simulink model "case3"  (R2024b)
settings: Solver=FixedStepAuto  StartTime=0  StopTime=1  FixedStep=1e-7  RelTol=1e-3
values from neighbouring files (symbols this model uses):
  SG_D_1_D = 0.01056    [IEEE9_case_parameters.m]    (also in case1_parameters.m; case2_parameters.m; case3_parameters.m; case4_parameters.m)
  SG_D_1_EnableSaturation = 0    [IEEE9_case_parameters.m]    (also in case1_parameters.m; case2_parameters.m; case3_parameters.m; case4_parameters.m)
  SG_D_1_f0 = 60    [IEEE9_case_parameters.m]    (also in case1_parameters.m; case2_parameters.m; case3_parameters.m; case4_parameters.m)
  SG_D_1_H = 7.5    [IEEE9_case_parameters.m]    (also in case1_parameters.m; case2_parameters.m; case3_parameters.m; case4_parameters.m)
  SG_D_1_K_A = 20    [IEEE9_case_parameters.m]    (also in case1_parameters.m; case2_parameters.m; case3_parameters.m; case4_parameters.m)
  SG_D_1_K_E = 1.000000e+1    (= 10)    [IEEE9_case_parameters.m]    (also in case1_parameters.m; case2_parameters.m; case3_parameters.m; case4_parameters.m)
  SG_D_1_K_F = 2.363    [IEEE9_case_parameters.m]    (also in case1_parameters.m; case2_parameters.m; case3_parameters.m; case4_parameters.m)
  SG_D_1_K_s = 0.5    [IEEE9_case_parameters.m]    (also in case1_parameters.m = 5; case2_parameters.m = 5; case3_parameters.m = 5; case4_parameters.m = 5)
  SG_D_1_R_a = 0.001088    [IEEE9_case_parameters.m]    (also in case1_parameters.m; case2_parameters.m; case3_parameters.m; case4_parameters.m)
  SG_D_1_S_A = 1    [IEEE9_case_parameters.m]    (also in case1_parameters.m; case2_parameters.m; case3_parameters.m; case4_parameters.m)
  SG_D_1_S_B = 0.103    [IEEE9_case_parameters.m]    (also in case1_parameters.m; case2_parameters.m; case3_parameters.m; case4_parameters.m)
  SG_D_1_S_N = 10.659857    [IEEE9_case_parameters.m]    (also in case1_parameters.m; case2_parameters.m; case3_parameters.m; case4_parameters.m)
  SG_D_1_SpeedPara = 200    [IEEE9_case_parameters.m]    (also in case1_parameters.m; case2_parameters.m; case3_parameters.m; case4_parameters.m)
  SG_D_1_T_0 = 0.720173    [IEEE9_case_parameters.m]    (also in case1_parameters.m = 0.755522; case2_parameters.m = 0.808931; case3_parameters.m = 0.869402; case4_parameters.m = 0.729316)
  SG_D_1_T_1 = 0.3    [IEEE9_case_parameters.m]    (also in case1_parameters.m; case2_parameters.m; case3_parameters.m; case4_parameters.m)
  SG_D_1_T_2 = 0.05    [IEEE9_case_parameters.m]    (also in case1_parameters.m; case2_parameters.m; case3_parameters.m; case4_parameters.m)
  SG_D_1_T_3 = 0.02    [IEEE9_case_parameters.m]    (also in case1_parameters.m; case2_parameters.m; case3_parameters.m; case4_parameters.m)
  SG_D_1_T_4 = 0.005    [IEEE9_case_parameters.m]    (also in case1_parameters.m; case2_parameters.m; case3_parameters.m; case4_parameters.m)
  SG_D_1_T_A = 0.02    [IEEE9_case_parameters.m]    (also in case1_parameters.m; case2_parameters.m; case3_parameters.m; case4_parameters.m)
  SG_D_1_T_dd = 8.000000e+0    (= 8)    [IEEE9_case_parameters.m]    (also in case1_parameters.m; case2_parameters.m; case3_parameters.m; case4_parameters.m)
  SG_D_1_T_ddd = 0.04    [IEEE9_case_parameters.m]    (also in case1_parameters.m; case2_parameters.m; case3_parameters.m; case4_parameters.m)
  SG_D_1_T_E = 0.314    [IEEE9_case_parameters.m]    (also in case1_parameters.m; case2_parameters.m; case3_parameters.m; case4_parameters.m)
  SG_D_1_T_F = 0.35    [IEEE9_case_parameters.m]    (also in case1_parameters.m; case2_parameters.m; case3_parameters.m; case4_parameters.m)
  SG_D_1_T_qd = 0.8    [IEEE9_case_parameters.m]    (also in case1_parameters.m; case2_parameters.m; case3_parameters.m; case4_parameters.m)
  SG_D_1_T_qdd = 0.02    [IEEE9_case_parameters.m]    (also in case1_parameters.m; case2_parameters.m; case3_parameters.m; case4_parameters.m)
  SG_D_1_T_speed = 0.1    [IEEE9_case_parameters.m]    (also in case1_parameters.m = 200; case2_parameters.m = 200; case3_parameters.m = 200; case4_parameters.m = 200)
  SG_D_1_T_w = 0.5    [IEEE9_case_parameters.m]    (also in case1_parameters.m; case2_parameters.m; case3_parameters.m; case4_parameters.m)
  SG_D_1_V_ref = 1.990276    [IEEE9_case_parameters.m]    (also in case1_parameters.m = 2.042296; case2_parameters.m = 2.051388; case3_parameters.m = 2.089584; case4_parameters.m = 2.01845)
  SG_D_1_w_ref = 376.991118    [IEEE9_case_parameters.m]    (also in case1_parameters.m; case2_parameters.m; case3_parameters.m; case4_parameters.m)
  SG_D_1_wb = 6.000000e+1    (= 60)    [IEEE9_case_parameters.m]    (also in case1_parameters.m; case2_parameters.m; case3_parameters.m; case4_parameters.m)
  SG_D_1_x_d = 1.9    [IEEE9_case_parameters.m]    (also in case1_parameters.m; case2_parameters.m; case3_parameters.m; case4_parameters.m)
  SG_D_1_x_dd = 0.302    [IEEE9_case_parameters.m]    (also in case1_parameters.m; case2_parameters.m; case3_parameters.m; case4_parameters.m)
  SG_D_1_x_ddd = 0.204    [IEEE9_case_parameters.m]    (also in case1_parameters.m; case2_parameters.m; case3_parameters.m; case4_parameters.m)
  SG_D_1_x_l = 0.05    [IEEE9_case_parameters.m]    (also in case1_parameters.m; case2_parameters.m; case3_parameters.m; case4_parameters.m)
  SG_D_1_x_q = 1.3    [IEEE9_case_parameters.m]    (also in case1_parameters.m; case2_parameters.m; case3_parameters.m; case4_parameters.m)
  SG_D_1_x_qd = 0.5    [IEEE9_case_parameters.m]    (also in case1_parameters.m; case2_parameters.m; case3_parameters.m; case4_parameters.m)
  SG_D_1_x_qdd = 0.3    [IEEE9_case_parameters.m]    (also in case1_parameters.m; case2_parameters.m; case3_parameters.m; case4_parameters.m)
  SG_D_2_D = 0.02    [IEEE9_case_parameters.m]    (also in case1_parameters.m; case2_parameters.m; case3_parameters.m; case4_parameters.m)
  SG_D_2_EnableSaturation = 0    [IEEE9_case_parameters.m]    (also in case1_parameters.m; case2_parameters.m; case3_parameters.m; case4_parameters.m)
  SG_D_2_f0 = 60    [IEEE9_case_parameters.m]    (also in case1_parameters.m; case2_parameters.m; case3_parameters.m; case4_parameters.m)
  SG_D_2_H = 8.000000e+0    (= 8)    [IEEE9_case_parameters.m]    (also in case1_parameters.m; case2_parameters.m; case3_parameters.m; case4_parameters.m)
  SG_D_2_K_A = 20    [IEEE9_case_parameters.m]    (also in case1_parameters.m; case2_parameters.m; case3_parameters.m; case4_parameters.m)
  SG_D_2_K_E = 1.000000e+1    (= 10)    [IEEE9_case_parameters.m]    (also in case1_parameters.m; case2_parameters.m; case3_parameters.m; case4_parameters.m)
  SG_D_2_K_F = 2.363    [IEEE9_case_parameters.m]    (also in case1_parameters.m; case2_parameters.m; case3_parameters.m; case4_parameters.m)
  SG_D_2_K_s = 0.5    [IEEE9_case_parameters.m]    (also in case1_parameters.m = 4; case2_parameters.m = 4; case3_parameters.m = 4; case4_parameters.m = 4)
  SG_D_2_R_a = 0.001088    [IEEE9_case_parameters.m]    (also in case1_parameters.m; case2_parameters.m; case3_parameters.m; case4_parameters.m)
  SG_D_2_S_A = 1    [IEEE9_case_parameters.m]    (also in case1_parameters.m; case2_parameters.m; case3_parameters.m; case4_parameters.m)
  SG_D_2_S_B = 0.103    [IEEE9_case_parameters.m]    (also in case1_parameters.m; case2_parameters.m; case3_parameters.m; case4_parameters.m)
  SG_D_2_S_N = 10.659857    [IEEE9_case_parameters.m]    (also in case1_parameters.m; case2_parameters.m; case3_parameters.m; case4_parameters.m)
  SG_D_2_SpeedPara = 200    [IEEE9_case_parameters.m]    (also in case1_parameters.m; case2_parameters.m; case3_parameters.m; case4_parameters.m)
  SG_D_2_T_0 = 1.632913    [IEEE9_case_parameters.m]    (also in case1_parameters.m = 1.632925; case2_parameters.m = 1.632915; case3_parameters.m = 1.632914; case4_parameters.m = 1.632927)
  SG_D_2_T_1 = 0.2    [IEEE9_case_parameters.m]    (also in case1_parameters.m; case2_parameters.m; case3_parameters.m; case4_parameters.m)
  SG_D_2_T_2 = 0.05    [IEEE9_case_parameters.m]    (also in case1_parameters.m; case2_parameters.m; case3_parameters.m; case4_parameters.m)
  SG_D_2_T_3 = 0.02    [IEEE9_case_parameters.m]    (also in case1_parameters.m; case2_parameters.m; case3_parameters.m; case4_parameters.m)
  SG_D_2_T_4 = 0.005    [IEEE9_case_parameters.m]    (also in case1_parameters.m; case2_parameters.m; case3_parameters.m; case4_parameters.m)
  SG_D_2_T_A = 0.02    [IEEE9_case_parameters.m]    (also in case1_parameters.m; case2_parameters.m; case3_parameters.m; case4_parameters.m)
  SG_D_2_T_dd = 7.9    [IEEE9_case_parameters.m]    (also in case1_parameters.m; case2_parameters.m; case3_parameters.m; case4_parameters.m)
  SG_D_2_T_ddd = 0.04    [IEEE9_case_parameters.m]    (also in case1_parameters.m; case2_parameters.m; case3_parameters.m; case4_parameters.m)
  SG_D_2_T_E = 0.314    [IEEE9_case_parameters.m]    (also in case1_parameters.m; case2_parameters.m; case3_parameters.m; case4_parameters.m)
  SG_D_2_T_F = 0.35    [IEEE9_case_parameters.m]    (also in case1_parameters.m; case2_parameters.m; case3_parameters.m; case4_parameters.m)
  SG_D_2_T_qd = 0.8    [IEEE9_case_parameters.m]    (also in case1_parameters.m; case2_parameters.m; case3_parameters.m; case4_parameters.m)
  SG_D_2_T_qdd = 0.015    [IEEE9_case_parameters.m]    (also in case1_parameters.m; case2_parameters.m; case3_parameters.m; case4_parameters.m)
  SG_D_2_T_speed = 0.1    [IEEE9_case_parameters.m]    (also in case1_parameters.m = 150; case2_parameters.m = 150; case3_parameters.m = 150; case4_parameters.m = 150)
  SG_D_2_T_w = 0.35    [IEEE9_case_parameters.m]    (also in case1_parameters.m; case2_parameters.m; case3_parameters.m; case4_parameters.m)
  SG_D_2_V_ref = 2.58547    [IEEE9_case_parameters.m]    (also in case1_parameters.m = 2.597896; case2_parameters.m = 2.587136; case3_parameters.m = 2.586042; case4_parameters.m = 2.599679)
  SG_D_2_w_ref = 376.991118    [IEEE9_case_parameters.m]    (also in case1_parameters.m; case2_parameters.m; case3_parameters.m; case4_parameters.m)
  SG_D_2_wb = 6.000000e+1    (= 60)    [IEEE9_case_parameters.m]    (also in case1_parameters.m; case2_parameters.m; case3_parameters.m; case4_parameters.m)
  SG_D_2_x_d = 1.8    [IEEE9_case_parameters.m]    (also in case1_parameters.m; case2_parameters.m; case3_parameters.m; case4_parameters.m)
  SG_D_2_x_dd = 0.302    [IEEE9_case_parameters.m]    (also in case1_parameters.m; case2_parameters.m; case3_parameters.m; case4_parameters.m)
  SG_D_2_x_ddd = 0.204    [IEEE9_case_parameters.m]    (also in case1_parameters.m; case2_parameters.m; case3_parameters.m; case4_parameters.m)
  SG_D_2_x_l = 0.05    [IEEE9_case_parameters.m]    (also in case1_parameters.m; case2_parameters.m; case3_parameters.m; case4_parameters.m)
  SG_D_2_x_q = 1.25    [IEEE9_case_parameters.m]    (also in case1_parameters.m; case2_parameters.m; case3_parameters.m; case4_parameters.m)
  SG_D_2_x_qd = 0.5    [IEEE9_case_parameters.m]    (also in case1_parameters.m; case2_parameters.m; case3_parameters.m; case4_parameters.m)
  SG_D_2_x_qdd = 0.3    [IEEE9_case_parameters.m]    (also in case1_parameters.m; case2_parameters.m; case3_parameters.m; case4_parameters.m)
  SG_D_3_D = 0.02    [IEEE9_case_parameters.m]    (also in case1_parameters.m; case2_parameters.m; case3_parameters.m; case4_parameters.m)
  SG_D_3_EnableSaturation = 0    [IEEE9_case_parameters.m]    (also in case1_parameters.m; case2_parameters.m; case3_parameters.m; case4_parameters.m)
  SG_D_3_f0 = 60    [IEEE9_case_parameters.m]    (also in case1_parameters.m; case2_parameters.m; case3_parameters.m; case4_parameters.m)
  SG_D_3_H = 7.7    [IEEE9_case_parameters.m]    (also in case1_parameters.m; case2_parameters.m; case3_parameters.m; case4_parameters.m)
  SG_D_3_K_A = 20    [IEEE9_case_parameters.m]    (also in case1_parameters.m; case2_parameters.m; case3_parameters.m; case4_parameters.m)
  SG_D_3_K_E = 1.000000e+1    (= 10)    [IEEE9_case_parameters.m]    (also in case1_parameters.m; case2_parameters.m; case3_parameters.m; case4_parameters.m)
  SG_D_3_K_F = 2.363    [IEEE9_case_parameters.m]    (also in case1_parameters.m; case2_parameters.m; case3_parameters.m; case4_parameters.m)
  SG_D_3_K_s = 0.2    [IEEE9_case_parameters.m]    (also in case1_parameters.m = 2; case2_parameters.m = 2; case3_parameters.m = 2; case4_parameters.m = 2)
  SG_D_3_R_a = 0.001088    [IEEE9_case_parameters.m]    (also in case1_parameters.m; case2_parameters.m; case3_parameters.m; case4_parameters.m)
  SG_D_3_S_A = 1    [IEEE9_case_parameters.m]    (also in case1_parameters.m; case2_parameters.m; case3_parameters.m; case4_parameters.m)
  SG_D_3_S_B = 0.103    [IEEE9_case_parameters.m]    (also in case1_parameters.m; case2_parameters.m; case3_parameters.m; case4_parameters.m)
  SG_D_3_S_N = 10.659857    [IEEE9_case_parameters.m]    (also in case1_parameters.m; case2_parameters.m; case3_parameters.m; case4_parameters.m)
  SG_D_3_SpeedPara = 200    [IEEE9_case_parameters.m]    (also in case1_parameters.m; case2_parameters.m; case3_parameters.m; case4_parameters.m)
  SG_D_3_T_0 = 0.850788    [IEEE9_case_parameters.m]    (also in case1_parameters.m = 0.850786; case2_parameters.m = 0.850787; case3_parameters.m; case4_parameters.m = 0.850786)
  SG_D_3_T_1 = 0.2    [IEEE9_case_parameters.m]    (also in case1_parameters.m; case2_parameters.m; case3_parameters.m; case4_parameters.m)
  SG_D_3_T_2 = 0.05    [IEEE9_case_parameters.m]    (also in case1_parameters.m; case2_parameters.m; case3_parameters.m; case4_parameters.m)
  SG_D_3_T_3 = 0.02    [IEEE9_case_parameters.m]    (also in case1_parameters.m; case2_parameters.m; case3_parameters.m; case4_parameters.m)
  SG_D_3_T_4 = 0.005    [IEEE9_case_parameters.m]    (also in case1_parameters.m; case2_parameters.m; case3_parameters.m; case4_parameters.m)
  SG_D_3_T_A = 0.02    [IEEE9_case_parameters.m]    (also in case1_parameters.m; case2_parameters.m; case3_parameters.m; case4_parameters.m)
  SG_D_3_T_dd = 8.1    [IEEE9_case_parameters.m]    (also in case1_parameters.m; case2_parameters.m; case3_parameters.m; case4_parameters.m)
  SG_D_3_T_ddd = 0.04    [IEEE9_case_parameters.m]    (also in case1_parameters.m; case2_parameters.m; case3_parameters.m; case4_parameters.m)
  SG_D_3_T_E = 0.314    [IEEE9_case_parameters.m]    (also in case1_parameters.m; case2_parameters.m; case3_parameters.m; case4_parameters.m)
  SG_D_3_T_F = 0.35    [IEEE9_case_parameters.m]    (also in case1_parameters.m; case2_parameters.m; case3_parameters.m; case4_parameters.m)
  SG_D_3_T_qd = 0.8    [IEEE9_case_parameters.m]    (also in case1_parameters.m; case2_parameters.m; case3_parameters.m; case4_parameters.m)
  SG_D_3_T_qdd = 0.015    [IEEE9_case_parameters.m]    (also in case1_parameters.m; case2_parameters.m; case3_parameters.m; case4_parameters.m)
  SG_D_3_T_speed = 0.1    [IEEE9_case_parameters.m]    (also in case1_parameters.m = 180; case2_parameters.m = 180; case3_parameters.m = 180; case4_parameters.m = 180)
  SG_D_3_T_w = 0.4    [IEEE9_case_parameters.m]    (also in case1_parameters.m; case2_parameters.m; case3_parameters.m; case4_parameters.m)
  SG_D_3_V_ref = 1.892727    [IEEE9_case_parameters.m]    (also in case1_parameters.m = 1.906439; case2_parameters.m = 1.895535; case3_parameters.m = 1.892105; case4_parameters.m = 1.906598)
  SG_D_3_w_ref = 376.991118    [IEEE9_case_parameters.m]    (also in case1_parameters.m; case2_parameters.m; case3_parameters.m; case4_parameters.m)
  SG_D_3_wb = 6.000000e+1    (= 60)    [IEEE9_case_parameters.m]    (also in case1_parameters.m; case2_parameters.m; case3_parameters.m; case4_parameters.m)
  SG_D_3_x_d = 1.85    [IEEE9_case_parameters.m]    (also in case1_parameters.m; case2_parameters.m; case3_parameters.m; case4_parameters.m)
  SG_D_3_x_dd = 0.302    [IEEE9_case_parameters.m]    (also in case1_parameters.m; case2_parameters.m; case3_parameters.m; case4_parameters.m)
  SG_D_3_x_ddd = 0.204    [IEEE9_case_parameters.m]    (also in case1_parameters.m; case2_parameters.m; case3_parameters.m; case4_parameters.m)
  SG_D_3_x_l = 0.05    [IEEE9_case_parameters.m]    (also in case1_parameters.m; case2_parameters.m; case3_parameters.m; case4_parameters.m)
  SG_D_3_x_q = 1.2    [IEEE9_case_parameters.m]    (also in case1_parameters.m; case2_parameters.m; case3_parameters.m; case4_parameters.m)
  SG_D_3_x_qd = 0.5    [IEEE9_case_parameters.m]    (also in case1_parameters.m; case2_parameters.m; case3_parameters.m; case4_parameters.m)
  SG_D_3_x_qdd = 0.3    [IEEE9_case_parameters.m]    (also in case1_parameters.m; case2_parameters.m; case3_parameters.m; case4_parameters.m)
(part 5 of 12)

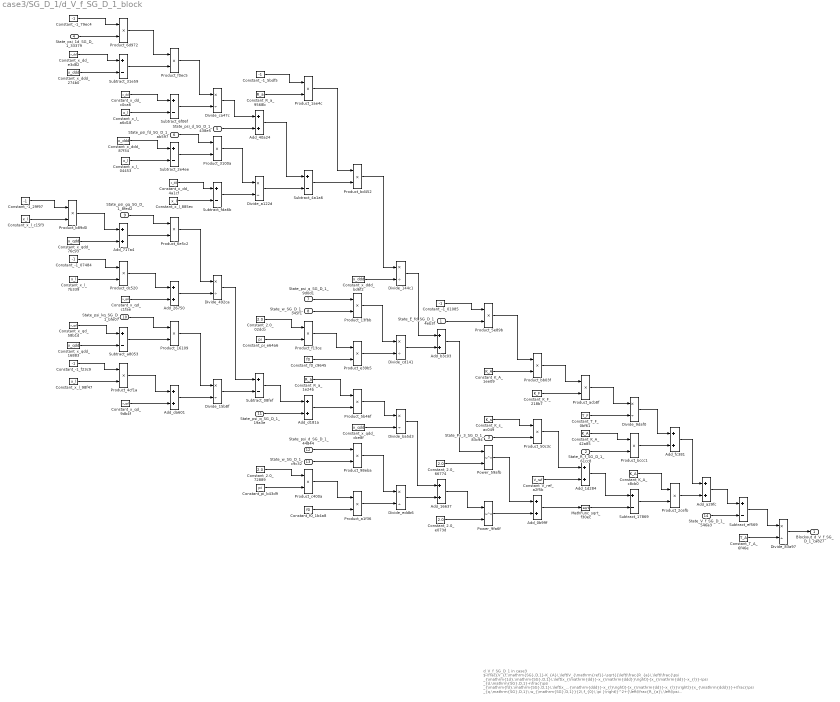
== system case3/SG_D_1/d_V_f_SG_D_1_block ==
  note: d_V_f_SG_D_1 in case3
      | $-\frac{V_{f,\mathrm{SG},D,1}-K_{A}\,\left(V_{\mathrm{ref}}-\sqrt{{\left(\frac{R_{a}\,\left(\frac{\psi _{\mathrm{1d},\mathrm{SG},D,1}\,\left(x_{\mathrm{dd}}-x_{\mathrm{ddd}}\right)}{x_{\mathrm{dd}}-x_{l}}-\psi _{d,\mathrm{SG},D,1}+\frac{\psi _{\mathrm{fd},\mathrm{SG},D,1}\,\left(x_{\mathrm{ddd}}-x_{l}\right)}{x_{\mathrm{dd}}-x_{l}}\right)}{x_{\mathrm{ddd}}}+\frac{\psi _{q,\mathrm{SG},D,1}\,w_{\mathrm{SG},D,1}}{2\,f_{0}\,\pi }\right)}^2+{\left(\frac{R_{a}\,\left(\psi _{q,\mathrm{SG},D,1}+\frac{\psi _{\mathrm{gq},\mathrm{SG},D,1}\,\left(x_{l}-x_{\mathrm{qdd}}\right)}{x_{l}-x_{\mathrm{qd}}}+\frac{\psi _{\mathrm{kq},\mathrm{SG},D,1}\,\left(x_{\mathrm{qd}}-x_{\mathrm{qdd}}\right)}{x_{l}-x_{\mathrm{qd}}}\right)}{x_{\mathrm{qdd}}}+\frac{\psi _{d,\mathrm{SG},D,1}\,w_{\mathrm{SG},D,1}}{2\,f_{0}\,\pi }\right)}^2}+K_{s}\,\mathrm{Px}_{3,\mathrm{SG},D,1}\right)-K_{A}\,R_{f,\mathrm{SG},D,1}+\frac{E_{\mathrm{fd},\mathrm{SG},D,1}\,K_{A}\,K_{F}}{T_{F}}}{T_{A}}$
      | Automatically generated on 2025-10-31 18:59:18 .
  State_E_fd_SG_D_1_4eb3f : Inport
  State_R_f_SG_D_1_61cc8 : Inport  Port=2
  State_Px_3_SG_D_1_83c94 : Inport  Port=3
  State_psi_1d_SG_D_1_33379 : Inport  Port=4
  State_psi_d_SG_D_1_438e5 : Inport  Port=5
  State_psi_fd_SG_D_1_ab597 : Inport  Port=6
  State_psi_q_SG_D_1_9d0d1 : Inport  Port=7
  State_w_SG_D_1_345f1 : Inport  Port=8
  State_psi_gq_SG_D_1_8fed2 : Inport  Port=9
  State_psi_kq_SG_D_1_bfe07 : Inport  Port=10
  State_psi_q_SG_D_1_19a3e : Inport  Port=11
  State_psi_d_SG_D_1_44844 : Inport  Port=12
  State_w_SG_D_1_c9c32 : Inport  Port=13
  State_V_f_SG_D_1_546a3 : Inport  Port=14
  Add_0b99f : Sum
  Add_16637 : Sum
  Add_1d284 : Sum
  Add_26750 : Sum
  Add_40a24 : Sum
  Add_717a4 : Sum
  Add_a29fc : Sum
  Add_b3c03 : Sum
  Add_d181a : Sum
  Add_da601 : Sum
  Add_fc381 : Sum
  Constant_-1_01085 : Constant  Value=-1
  Constant_-1_07484 : Constant  Value=-1
  Constant_-1_29f97 : Constant  Value=-1
  Constant_-1_5bdf5 : Constant  Value=-1
  Constant_-1_79ec4 : Constant  Value=-1
  Constant_-1_f23c9 : Constant  Value=-1
  Constant_2.0_02dcb : Constant  Value=2.0
  Constant_2.0_66774 : Constant  Value=2.0
  Constant_2.0_72889 : Constant  Value=2.0
  Constant_2.0_e073d : Constant  Value=2.0
  Constant_K_A_1ee09 : Constant  Value=K_A
  Constant_K_A_42a85 : Constant  Value=K_A
  Constant_K_A_c8cb0 : Constant  Value=K_A
  Constant_K_F_218b7 : Constant  Value=K_F
  Constant_K_s_ac049 : Constant  Value=K_s
  Constant_R_a_1e24b : Constant  Value=R_a
  Constant_R_a_9568b : Constant  Value=R_a
  Constant_T_A_6f46e : Constant  Value=T_A
  Constant_T_F_0bf61 : Constant  Value=T_F
  Constant_V_ref_a2f5b : Constant  Value=V_ref
  Constant_f0_1b4a8 : Constant  Value=f0
  Constant_f0_c9645 : Constant  Value=f0
  Constant_pi_b43d9 : Constant  Value=pi
  Constant_pi_e64a6 : Constant  Value=pi
  Constant_x_dd_4a1cf : Constant  Value=x_dd
  Constant_x_dd_c0ca6 : Constant  Value=x_dd
  Constant_x_dd_e3d82 : Constant  Value=x_dd
  Constant_x_ddd_274b0 : Constant  Value=x_ddd
  Constant_x_ddd_87f34 : Constant  Value=x_ddd
  Constant_x_ddd_bd6f2 : Constant  Value=x_ddd
  Constant_x_l_04453 : Constant  Value=x_l
  Constant_x_l_7b339 : Constant  Value=x_l
  Constant_x_l_885ec : Constant  Value=x_l
  Constant_x_l_98f47 : Constant  Value=x_l
  Constant_x_l_a6d18 : Constant  Value=x_l
  Constant_x_l_c15f3 : Constant  Value=x_l
  Constant_x_qd_58b1d : Constant  Value=x_qd
  Constant_x_qd_9db4f : Constant  Value=x_qd
  Constant_x_qd_c1fae : Constant  Value=x_qd
  Constant_x_qdd_16883 : Constant  Value=x_qdd
  Constant_x_qdd_76c93 : Constant  Value=x_qdd
  Constant_x_qdd_dce8f : Constant  Value=x_qdd
  Divide_144c1 : Product  Inputs=*/
  Divide_15b8f : Product  Inputs=*/
  Divide_492ca : Product  Inputs=*/
  Divide_83a97 : Product  Inputs=*/
  Divide_9daf0 : Product  Inputs=*/
  Divide_a122d : Product  Inputs=*/
  Divide_ba5d3 : Product  Inputs=*/
  Divide_ca47c : Product  Inputs=*/
  Divide_cd141 : Product  Inputs=*/
  Divide_eddb6 : Product  Inputs=*/
  MathFunc_sqrt_f30ec : Sqrt
  Power_59afb : Math  Operator=pow
  Power_9fa6f : Math  Operator=pow
  Product_13fbb : Product
  Product_16109 : Product
  Product_1ae4c : Product
  Product_2cefb : Product
  Product_3100a : Product
  Product_4cf1a : Product
  Product_50c3c : Product
  Product_5b46f : Product
  Product_5e89b : Product
  Product_6d972 : Product
  Product_6e5c2 : Product
  Product_98eba : Product
  Product_a1f36 : Product
  Product_acb8f : Product
  Product_b89d0 : Product
  Product_bb03f : Product
  Product_bccc1 : Product
  Product_bd452 : Product
  Product_c400a : Product
  Product_dc520 : Product
  Product_e39b5 : Product
  Product_f0ec5 : Product
  Product_f13ce : Product
  Subtract_08fef : Sum  Inputs=+-
  Subtract_17869 : Sum  Inputs=+-
  Subtract_2e4ee : Sum  Inputs=+-
  Subtract_31e59 : Sum  Inputs=+-
  Subtract_4a1a6 : Sum  Inputs=+-
  Subtract_6f06f : Sum  Inputs=+-
  Subtract_a8053 : Sum  Inputs=+-
  Subtract_ef569 : Sum  Inputs=+-
  Subtract_fda6b : Sum  Inputs=+-
  Blockout_d_V_f_SG_D_1_ca827 : Outport
  wires:
  Constant_-1_f23c9/1 -> Product_4cf1a/1
  Constant_-1_29f97/1 -> Product_b89d0/1
  State_psi_d_SG_D_1_44844/1 -> Product_98eba/1
  Constant_x_qd_9db4f/1 -> Add_da601/2
  Constant_x_qdd_76c93/1 -> Add_717a4/2
  State_w_SG_D_1_c9c32/1 -> Product_98eba/2
  Constant_x_l_c15f3/1 -> Product_b89d0/2
  Subtract_4a1a6/1 -> Product_bd452/2
  Constant_x_l_98f47/1 -> Product_4cf1a/2
  Constant_x_dd_e3d82/1 -> Subtract_31e59/1
  Constant_R_a_9568b/1 -> Product_1ae4c/2
  Constant_-1_79ec4/1 -> Product_6d972/1
  Divide_a122d/1 -> Subtract_4a1a6/2
  Constant_x_ddd_274b0/1 -> Subtract_31e59/2
  Add_da601/1 -> Divide_15b8f/2
  State_psi_1d_SG_D_1_33379/1 -> Product_6d972/2
  Add_26750/1 -> Divide_492ca/2
  Subtract_a8053/1 -> Product_16109/2
  Product_acb8f/1 -> Divide_9daf0/1
  Product_f13ce/1 -> Product_e39b5/1
  Product_b89d0/1 -> Add_717a4/1
  Constant_-1_07484/1 -> Product_dc520/1
  Constant_x_l_7b339/1 -> Product_dc520/2
  Add_40a24/1 -> Subtract_4a1a6/1
  Constant_2.0_72889/1 -> Product_c400a/1
  Constant_x_qd_58b1d/1 -> Subtract_a8053/1
  Product_6d972/1 -> Product_f0ec5/1
  Constant_pi_b43d9/1 -> Product_c400a/2
  Constant_x_qdd_16883/1 -> Subtract_a8053/2
  Subtract_31e59/1 -> Product_f0ec5/2
  State_psi_q_SG_D_1_19a3e/1 -> Add_d181a/2
  Constant_x_dd_c0ca6/1 -> Subtract_6f06f/1
  Constant_x_l_a6d18/1 -> Subtract_6f06f/2
  Constant_x_ddd_87f34/1 -> Subtract_2e4ee/1
  Constant_x_l_04453/1 -> Subtract_2e4ee/2
  State_psi_gq_SG_D_1_8fed2/1 -> Product_6e5c2/1
  Add_717a4/1 -> Product_6e5c2/2
  Product_dc520/1 -> Add_26750/1
  Constant_x_qd_c1fae/1 -> Add_26750/2
  Divide_ca47c/1 -> Add_40a24/1
  Subtract_6f06f/1 -> Divide_ca47c/2
  State_psi_kq_SG_D_1_bfe07/1 -> Product_16109/1
  Divide_83a97/1 -> Blockout_d_V_f_SG_D_1_ca827/1
  Product_4cf1a/1 -> Add_da601/1
  Product_f0ec5/1 -> Divide_ca47c/1
  State_psi_fd_SG_D_1_ab597/1 -> Product_3100a/1
  State_w_SG_D_1_345f1/1 -> Product_13fbb/2
  Subtract_2e4ee/1 -> Product_3100a/2
  Constant_x_dd_4a1cf/1 -> Subtract_fda6b/1
  Constant_x_l_885ec/1 -> Subtract_fda6b/2
  Product_6e5c2/1 -> Divide_492ca/1
  Product_1ae4c/1 -> Product_bd452/1
  Product_16109/1 -> Divide_15b8f/1
  State_psi_d_SG_D_1_438e5/1 -> Add_40a24/2
  Product_3100a/1 -> Divide_a122d/1
  Subtract_fda6b/1 -> Divide_a122d/2
  Divide_492ca/1 -> Subtract_08fef/1
  Divide_15b8f/1 -> Subtract_08fef/2
  Constant_-1_5bdf5/1 -> Product_1ae4c/1
  Constant_2.0_02dcb/1 -> Product_f13ce/1
  Constant_pi_e64a6/1 -> Product_f13ce/2
  Subtract_08fef/1 -> Add_d181a/1
  State_psi_q_SG_D_1_9d0d1/1 -> Product_13fbb/1
  Constant_f0_c9645/1 -> Product_e39b5/2
  Constant_R_a_1e24b/1 -> Product_5b46f/1
  Add_d181a/1 -> Product_5b46f/2
  Product_c400a/1 -> Product_a1f36/1
  Power_59afb/1 -> Add_0b99f/1
  Constant_f0_1b4a8/1 -> Product_a1f36/2
  Product_bd452/1 -> Divide_144c1/1
  Constant_x_ddd_bd6f2/1 -> Divide_144c1/2
  Product_13fbb/1 -> Divide_cd141/1
  Product_e39b5/1 -> Divide_cd141/2
  Product_5b46f/1 -> Divide_ba5d3/1
  Constant_x_qdd_dce8f/1 -> Divide_ba5d3/2
  Product_98eba/1 -> Divide_eddb6/1
  Product_a1f36/1 -> Divide_eddb6/2
  Divide_144c1/1 -> Add_b3c03/1
  Divide_cd141/1 -> Add_b3c03/2
  Divide_ba5d3/1 -> Add_16637/1
  Divide_eddb6/1 -> Add_16637/2
  Constant_-1_01085/1 -> Product_5e89b/1
  State_E_fd_SG_D_1_4eb3f/1 -> Product_5e89b/2
  Add_b3c03/1 -> Power_59afb/1
  Constant_2.0_66774/1 -> Power_59afb/2
  Add_16637/1 -> Power_9fa6f/1
  Constant_2.0_e073d/1 -> Power_9fa6f/2
  Product_5e89b/1 -> Product_bb03f/1
  Constant_K_A_1ee09/1 -> Product_bb03f/2
  Constant_K_s_ac049/1 -> Product_50c3c/1
  State_Px_3_SG_D_1_83c94/1 -> Product_50c3c/2
  Power_9fa6f/1 -> Add_0b99f/2
  Divide_9daf0/1 -> Add_fc381/1
  Product_bb03f/1 -> Product_acb8f/1
  Constant_K_F_218b7/1 -> Product_acb8f/2
  Product_50c3c/1 -> Add_1d284/1
  Constant_V_ref_a2f5b/1 -> Add_1d284/2
  Add_0b99f/1 -> MathFunc_sqrt_f30ec/1
  Constant_T_F_0bf61/1 -> Divide_9daf0/2
  Constant_K_A_42a85/1 -> Product_bccc1/1
  State_R_f_SG_D_1_61cc8/1 -> Product_bccc1/2
  Add_1d284/1 -> Subtract_17869/1
  MathFunc_sqrt_f30ec/1 -> Subtract_17869/2
  Constant_T_A_6f46e/1 -> Divide_83a97/2
  Product_bccc1/1 -> Add_fc381/2
  Constant_K_A_c8cb0/1 -> Product_2cefb/1
  Subtract_17869/1 -> Product_2cefb/2
  Add_fc381/1 -> Add_a29fc/1
  Product_2cefb/1 -> Add_a29fc/2
  Add_a29fc/1 -> Subtract_ef569/1
  State_V_f_SG_D_1_546a3/1 -> Subtract_ef569/2
  Subtract_ef569/1 -> Divide_83a97/1

== system case3/SG_D_1/d_psi_1d_SG_D_1_block ==
  note: d_psi_1d_SG_D_1 in case3
      | $-\frac{\psi _{\mathrm{1d},\mathrm{SG},D,1}-\psi _{\mathrm{fd},\mathrm{SG},D,1}+\frac{\left(x_{\mathrm{dd}}-x_{l}\right)\,\left(\frac{\psi _{\mathrm{1d},\mathrm{SG},D,1}\,\left(x_{\mathrm{dd}}-x_{\mathrm{ddd}}\right)}{x_{\mathrm{dd}}-x_{l}}-\psi _{d,\mathrm{SG},D,1}+\frac{\psi _{\mathrm{fd},\mathrm{SG},D,1}\,\left(x_{\mathrm{ddd}}-x_{l}\right)}{x_{\mathrm{dd}}-x_{l}}\right)}{x_{\mathrm{ddd}}}}{T_{\mathrm{ddd}}}$
      | Automatically generated on 2025-10-31 18:58:53 .
  State_psi_1d_SG_D_1_e272b : Inport
  State_psi_fd_SG_D_1_fedb2 : Inport  Port=2
  State_psi_1d_SG_D_1_7d194 : Inport  Port=3
  State_psi_d_SG_D_1_96939 : Inport  Port=4
  State_psi_fd_SG_D_1_95a16 : Inport  Port=5
  Add_42b21 : Sum
  Add_5d8a9 : Sum
  Add_dc4dc : Sum
  Constant_-1_e75cf : Constant  Value=-1
  Constant_-1_f7b2a : Constant  Value=-1
  Constant_T_ddd_a102f : Constant  Value=T_ddd
  Constant_x_dd_0e29c : Constant  Value=x_dd
  Constant_x_dd_79a01 : Constant  Value=x_dd
  Constant_x_dd_a89d7 : Constant  Value=x_dd
  Constant_x_dd_ae813 : Constant  Value=x_dd
  Constant_x_ddd_54350 : Constant  Value=x_ddd
  Constant_x_ddd_db1e2 : Constant  Value=x_ddd
  Constant_x_ddd_ec4a0 : Constant  Value=x_ddd
  Constant_x_l_0d07e : Constant  Value=x_l
  Constant_x_l_3bc90 : Constant  Value=x_l
  Constant_x_l_98e07 : Constant  Value=x_l
  Constant_x_l_a3c04 : Constant  Value=x_l
  Divide_7d352 : Product  Inputs=*/
  Divide_7d7e2 : Product  Inputs=*/
  Divide_835f4 : Product  Inputs=*/
  Divide_8fc52 : Product  Inputs=*/
  Product_4abd4 : Product
  Product_56b10 : Product
  Product_79689 : Product
  Product_afc20 : Product
  Product_ca7ac : Product
  Subtract_0badf : Sum  Inputs=+-
  Subtract_167cf : Sum  Inputs=+-
  Subtract_19f3a : Sum  Inputs=+-
  Subtract_6cf58 : Sum  Inputs=+-
  Subtract_f73bd : Sum  Inputs=+-
  Subtract_f8e45 : Sum  Inputs=+-
  Blockout_d_psi_1d_SG_D_1_9d8e2 : Outport
  wires:
  Product_79689/1 -> Product_56b10/1
  Constant_-1_f7b2a/1 -> Product_79689/1
  Subtract_19f3a/1 -> Product_56b10/2
  State_psi_1d_SG_D_1_7d194/1 -> Product_79689/2
  Subtract_167cf/1 -> Product_afc20/1
  State_psi_d_SG_D_1_96939/1 -> Add_dc4dc/2
  Constant_x_dd_0e29c/1 -> Subtract_6cf58/1
  Constant_x_l_98e07/1 -> Subtract_167cf/2
  Constant_x_dd_79a01/1 -> Subtract_19f3a/1
  Subtract_0badf/1 -> Product_4abd4/2
  Constant_x_l_a3c04/1 -> Subtract_6cf58/2
  Divide_835f4/1 -> Subtract_f8e45/2
  Constant_x_ddd_db1e2/1 -> Subtract_19f3a/2
  Constant_x_ddd_54350/1 -> Subtract_0badf/1
  Constant_x_l_3bc90/1 -> Subtract_0badf/2
  Add_5d8a9/1 -> Add_42b21/1
  Product_56b10/1 -> Divide_8fc52/1
  Divide_7d352/1 -> Add_42b21/2
  Subtract_6cf58/1 -> Divide_8fc52/2
  State_psi_fd_SG_D_1_95a16/1 -> Product_4abd4/1
  Constant_x_dd_a89d7/1 -> Subtract_f73bd/1
  Constant_x_l_0d07e/1 -> Subtract_f73bd/2
  Constant_x_ddd_ec4a0/1 -> Divide_7d352/2
  Subtract_f8e45/1 -> Product_afc20/2
  Divide_8fc52/1 -> Add_dc4dc/1
  Product_4abd4/1 -> Divide_835f4/1
  Subtract_f73bd/1 -> Divide_835f4/2
  Product_afc20/1 -> Divide_7d352/1
  Constant_x_dd_ae813/1 -> Subtract_167cf/1
  Add_dc4dc/1 -> Subtract_f8e45/1
  Constant_-1_e75cf/1 -> Product_ca7ac/1
  State_psi_1d_SG_D_1_e272b/1 -> Product_ca7ac/2
  Product_ca7ac/1 -> Add_5d8a9/1
  State_psi_fd_SG_D_1_fedb2/1 -> Add_5d8a9/2
  Add_42b21/1 -> Divide_7d7e2/1
  Constant_T_ddd_a102f/1 -> Divide_7d7e2/2
  Divide_7d7e2/1 -> Blockout_d_psi_1d_SG_D_1_9d8e2/1

== system case3/SG_D_1/d_psi_d_SG_D_1_block ==
  note: d_psi_d_SG_D_1 in case3
      | $2\,\pi \,f_{0}\,\left(v_{d,\mathrm{SG},D,1}\,\sin\left(\theta _{\mathrm{SG},D,1}\right)-v_{q,\mathrm{SG},D,1}\,\cos\left(\theta _{\mathrm{SG},D,1}\right)+\frac{R_{a}\,\left(\frac{\psi _{\mathrm{1d},\mathrm{SG},D,1}\,\left(x_{\mathrm{dd}}-x_{\mathrm{ddd}}\right)}{x_{\mathrm{dd}}-x_{l}}-\psi _{d,\mathrm{SG},D,1}+\frac{\psi _{\mathrm{fd},\mathrm{SG},D,1}\,\left(x_{\mathrm{ddd}}-x_{l}\right)}{x_{\mathrm{dd}}-x_{l}}\right)}{x_{\mathrm{ddd}}}+\frac{\psi _{q,\mathrm{SG},D,1}\,w_{\mathrm{SG},D,1}}{2\,f_{0}\,\pi }\right)$
      | Automatically generated on 2025-10-31 18:58:24 .
  State_psi_1d_SG_D_1_32408 : Inport
  State_psi_d_SG_D_1_ff70f : Inport  Port=2
  State_psi_fd_SG_D_1_dc6ee : Inport  Port=3
  Input_v_d_SG_D_1_d8586 : Inport  Port=4
  State_theta_SG_D_1_f81ae : Inport  Port=5
  Input_v_q_SG_D_1_8ffea : Inport  Port=6
  State_theta_SG_D_1_ab80e : Inport  Port=7
  State_psi_q_SG_D_1_46dab : Inport  Port=8
  State_w_SG_D_1_754af : Inport  Port=9
  Add_8f8b7 : Sum
  Add_b6504 : Sum
  Constant_-1_35ea6 : Constant  Value=-1
  Constant_-2.0_006e7 : Constant  Value=-2.0
  Constant_2.0_73bad : Constant  Value=2.0
  Constant_R_a_94202 : Constant  Value=R_a
  Constant_f0_7312d : Constant  Value=f0
  Constant_f0_bd640 : Constant  Value=f0
  Constant_pi_4a685 : Constant  Value=pi
  Constant_pi_f9cc3 : Constant  Value=pi
  Constant_x_dd_5e46c : Constant  Value=x_dd
  Constant_x_dd_bd345 : Constant  Value=x_dd
  Constant_x_dd_e356b : Constant  Value=x_dd
  Constant_x_ddd_264fd : Constant  Value=x_ddd
  Constant_x_ddd_7c458 : Constant  Value=x_ddd
  Constant_x_ddd_8936d : Constant  Value=x_ddd
  Constant_x_l_071d9 : Constant  Value=x_l
  Constant_x_l_878fd : Constant  Value=x_l
  Constant_x_l_94d8d : Constant  Value=x_l
  Divide_2ef13 : Product  Inputs=*/
  Divide_43845 : Product  Inputs=*/
  Divide_5ee37 : Product  Inputs=*/
  Divide_79d51 : Product  Inputs=*/
  MathFunc_cos_d08ba : Trigonometry  Operator=cos
  MathFunc_sin_56f8d : Trigonometry
  Product_25090 : Product
  Product_656d1 : Product
  Product_6e197 : Product
  Product_7d821 : Product
  Product_7fae8 : Product
  Product_83d36 : Product
  Product_a0b6a : Product
  Product_a589e : Product
  Product_a72cc : Product
  Product_d6dec : Product
  Product_e3501 : Product
  Product_ef419 : Product
  Subtract_3a625 : Sum  Inputs=+-
  Subtract_40248 : Sum  Inputs=+-
  Subtract_59c15 : Sum  Inputs=+-
  Subtract_7bf87 : Sum  Inputs=+-
  Subtract_8b523 : Sum  Inputs=+-
  Subtract_c1886 : Sum  Inputs=+-
  Subtract_c1d19 : Sum  Inputs=+-
  Blockout_d_psi_d_SG_D_1_c7dc2 : Outport
  wires:
  Add_b6504/1 -> Subtract_3a625/1
  Product_ef419/1 -> Divide_2ef13/1
  Subtract_c1886/1 -> Product_ef419/2
  Divide_2ef13/1 -> Add_b6504/1
  Product_a72cc/1 -> Product_ef419/1
  Constant_x_ddd_7c458/1 -> Subtract_c1886/2
  Constant_x_dd_bd345/1 -> Subtract_c1886/1
  State_psi_1d_SG_D_1_32408/1 -> Product_a72cc/2
  Constant_-1_35ea6/1 -> Product_a72cc/1
  Product_e3501/1 -> Divide_43845/1
  Constant_x_l_878fd/1 -> Subtract_59c15/2
  State_psi_d_SG_D_1_ff70f/1 -> Add_b6504/2
  Constant_x_dd_e356b/1 -> Subtract_59c15/1
  Constant_x_ddd_8936d/1 -> Subtract_7bf87/1
  Constant_x_l_94d8d/1 -> Subtract_7bf87/2
  Subtract_59c15/1 -> Divide_2ef13/2
  State_psi_fd_SG_D_1_dc6ee/1 -> Product_e3501/1
  Constant_x_ddd_264fd/1 -> Divide_5ee37/2
  Subtract_7bf87/1 -> Product_e3501/2
  Product_6e197/1 -> Subtract_40248/2
  Constant_x_dd_5e46c/1 -> Subtract_8b523/1
  Constant_x_l_071d9/1 -> Subtract_8b523/2
  Subtract_8b523/1 -> Divide_43845/2
  Divide_43845/1 -> Subtract_3a625/2
  Constant_R_a_94202/1 -> Product_83d36/1
  Subtract_3a625/1 -> Product_83d36/2
  MathFunc_cos_d08ba/1 -> Product_7fae8/2
  State_theta_SG_D_1_f81ae/1 -> MathFunc_sin_56f8d/1
  Divide_5ee37/1 -> Subtract_40248/1
  Product_83d36/1 -> Divide_5ee37/1
  MathFunc_sin_56f8d/1 -> Product_6e197/2
  Input_v_d_SG_D_1_d8586/1 -> Product_6e197/1
  Product_656d1/1 -> Blockout_d_psi_d_SG_D_1_c7dc2/1
  Product_d6dec/1 -> Product_656d1/1
  Product_a0b6a/1 -> Product_d6dec/1
  State_theta_SG_D_1_ab80e/1 -> MathFunc_cos_d08ba/1
  Constant_2.0_73bad/1 -> Product_a589e/1
  Constant_pi_4a685/1 -> Product_a589e/2
  Input_v_q_SG_D_1_8ffea/1 -> Product_7fae8/1
  Constant_f0_7312d/1 -> Product_d6dec/2
  State_psi_q_SG_D_1_46dab/1 -> Product_7d821/1
  State_w_SG_D_1_754af/1 -> Product_7d821/2
  Product_a589e/1 -> Product_25090/1
  Constant_pi_f9cc3/1 -> Product_a0b6a/2
  Constant_f0_bd640/1 -> Product_25090/2
  Constant_-2.0_006e7/1 -> Product_a0b6a/1
  Add_8f8b7/1 -> Subtract_c1d19/1
  Subtract_40248/1 -> Add_8f8b7/1
  Product_7fae8/1 -> Add_8f8b7/2
  Product_7d821/1 -> Divide_79d51/1
  Product_25090/1 -> Divide_79d51/2
  Divide_79d51/1 -> Subtract_c1d19/2
  Subtract_c1d19/1 -> Product_656d1/2

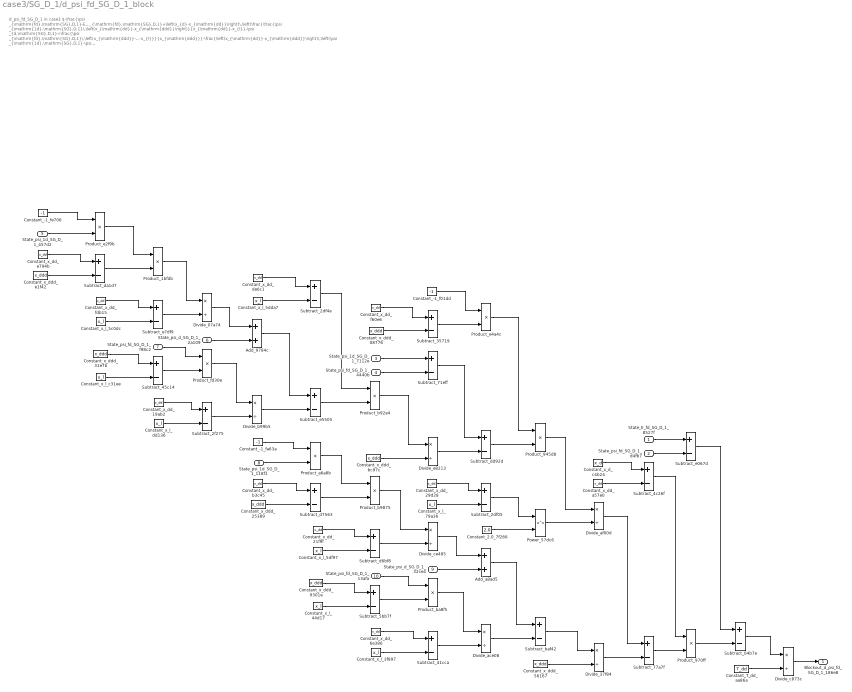
== system case3/SG_D_1/d_psi_fd_SG_D_1_block ==
  note: d_psi_fd_SG_D_1 in case3
      | $-\frac{\psi _{\mathrm{fd},\mathrm{SG},D,1}-E_{\mathrm{fd},\mathrm{SG},D,1}+\left(x_{d}-x_{\mathrm{dd}}\right)\,\left(\frac{\frac{\psi _{\mathrm{1d},\mathrm{SG},D,1}\,\left(x_{\mathrm{dd}}-x_{\mathrm{ddd}}\right)}{x_{\mathrm{dd}}-x_{l}}-\psi _{d,\mathrm{SG},D,1}+\frac{\psi _{\mathrm{fd},\mathrm{SG},D,1}\,\left(x_{\mathrm{ddd}}-x_{l}\right)}{x_{\mathrm{dd}}-x_{l}}}{x_{\mathrm{ddd}}}-\frac{\left(x_{\mathrm{dd}}-x_{\mathrm{ddd}}\right)\,\left(\psi _{\mathrm{1d},\mathrm{SG},D,1}-\psi _{\mathrm{fd},\mathrm{SG},D,1}+\frac{\left(x_{\mathrm{dd}}-x_{l}\right)\,\left(\frac{\psi _{\mathrm{1d},\mathrm{SG},D,1}\,\left(x_{\mathrm{dd}}-x_{\mathrm{ddd}}\right)}{x_{\mathrm{dd}}-x_{l}}-\psi _{d,\mathrm{SG},D,1}+\frac{\psi _{\mathrm{fd},\mathrm{SG},D,1}\,\left(x_{\mathrm{ddd}}-x_{l}\right)}{x_{\mathrm{dd}}-x_{l}}\right)}{x_{\mathrm{ddd}}}\right)}{{\left(x_{\mathrm{dd}}-x_{l}\right)}^2}\right)}{T_{\mathrm{dd}}}$
      | Automatically generated on 2025-10-31 18:58:50 .
  State_E_fd_SG_D_1_8527f : Inport
  State_psi_fd_SG_D_1_d4fb7 : Inport  Port=2
  State_psi_1d_SG_D_1_7112e : Inport  Port=3
  State_psi_fd_SG_D_1_4440b : Inport  Port=4
  State_psi_1d_SG_D_1_457d2 : Inport  Port=5
  State_psi_d_SG_D_1_2a109 : Inport  Port=6
  State_psi_fd_SG_D_1_f98c2 : Inport  Port=7
  State_psi_1d_SG_D_1_118f1 : Inport  Port=8
  State_psi_d_SG_D_1_32ce4 : Inport  Port=9
  State_psi_fd_SG_D_1_13afa : Inport  Port=10
  Add_9784c : Sum
  Add_a8ad5 : Sum
  Constant_-1_f01dd : Constant  Value=-1
  Constant_-1_fa63a : Constant  Value=-1
  Constant_-1_fe706 : Constant  Value=-1
  Constant_2.0_7f266 : Constant  Value=2.0
  Constant_T_dd_aa86a : Constant  Value=T_dd
  Constant_x_d_c4b24 : Constant  Value=x_d
  Constant_x_dd_19ab2 : Constant  Value=x_dd
  Constant_x_dd_21f9f : Constant  Value=x_dd
  Constant_x_dd_29d28 : Constant  Value=x_dd
  Constant_x_dd_6e386 : Constant  Value=x_dd
  Constant_x_dd_a57e0 : Constant  Value=x_dd
  Constant_x_dd_b3c45 : Constant  Value=x_dd
  Constant_x_dd_de6c1 : Constant  Value=x_dd
  Constant_x_dd_e794b : Constant  Value=x_dd
  Constant_x_dd_f60e6 : Constant  Value=x_dd
  Constant_x_dd_fdb15 : Constant  Value=x_dd
  Constant_x_ddd_08776 : Constant  Value=x_ddd
  Constant_x_ddd_25389 : Constant  Value=x_ddd
  Constant_x_ddd_31e7b : Constant  Value=x_ddd
  Constant_x_ddd_56167 : Constant  Value=x_ddd
  Constant_x_ddd_9301e : Constant  Value=x_ddd
  Constant_x_ddd_bc97c : Constant  Value=x_ddd
  Constant_x_ddd_e1f42 : Constant  Value=x_ddd
  Constant_x_l_3f897 : Constant  Value=x_l
  Constant_x_l_44d17 : Constant  Value=x_l
  Constant_x_l_5c0dc : Constant  Value=x_l
  Constant_x_l_5dda7 : Constant  Value=x_l
  Constant_x_l_5df97 : Constant  Value=x_l
  Constant_x_l_79a36 : Constant  Value=x_l
  Constant_x_l_c31ee : Constant  Value=x_l
  Constant_x_l_dd136 : Constant  Value=x_l
  Divide_07a74 : Product  Inputs=*/
  Divide_37f84 : Product  Inputs=*/
  Divide_ace08 : Product  Inputs=*/
  Divide_af00d : Product  Inputs=*/
  Divide_b99b5 : Product  Inputs=*/
  Divide_c873c : Product  Inputs=*/
  Divide_ce485 : Product  Inputs=*/
  Divide_e8213 : Product  Inputs=*/
  Power_57dc6 : Math  Operator=pow
  Product_1bfdb : Product
  Product_945d8 : Product
  Product_970ff : Product
  Product_a6a8b : Product
  Product_b92e4 : Product
  Product_b9875 : Product
  Product_ba8f5 : Product
  Product_e2f9b : Product
  Product_e4a4c : Product
  Product_fd30e : Product
  Subtract_04b7e : Sum  Inputs=+-
  Subtract_2df05 : Sum  Inputs=+-
  Subtract_2df4e : Sum  Inputs=+-
  Subtract_2f275 : Sum  Inputs=+-
  Subtract_35719 : Sum  Inputs=+-
  Subtract_41cca : Sum  Inputs=+-
  Subtract_45c14 : Sum  Inputs=+-
  Subtract_4c26f : Sum  Inputs=+-
  Subtract_5bb7f : Sum  Inputs=+-
  Subtract_71eff : Sum  Inputs=+-
  Subtract_77a7f : Sum  Inputs=+-
  Subtract_baf42 : Sum  Inputs=+-
  Subtract_d6bf8 : Sum  Inputs=+-
  Subtract_d7563 : Sum  Inputs=+-
  Subtract_da1d7 : Sum  Inputs=+-
  Subtract_dd92d : Sum  Inputs=+-
  Subtract_e067d : Sum  Inputs=+-
  Subtract_e5505 : Sum  Inputs=+-
  Subtract_e7df9 : Sum  Inputs=+-
  Blockout_d_psi_fd_SG_D_1_186e8 : Outport
  wires:
  State_psi_d_SG_D_1_2a109/1 -> Add_9784c/2
  Constant_x_dd_fdb15/1 -> Subtract_e7df9/1
  Product_1bfdb/1 -> Divide_07a74/1
  Subtract_da1d7/1 -> Product_1bfdb/2
  Subtract_e5505/1 -> Product_b92e4/2
  Product_e2f9b/1 -> Product_1bfdb/1
  Constant_x_dd_e794b/1 -> Subtract_da1d7/1
  Constant_x_l_5dda7/1 -> Subtract_2df4e/2
  Constant_-1_fe706/1 -> Product_e2f9b/1
  Subtract_2df4e/1 -> Product_b92e4/1
  Constant_x_l_5c0dc/1 -> Subtract_e7df9/2
  Constant_x_ddd_e1f42/1 -> Subtract_da1d7/2
  State_psi_1d_SG_D_1_457d2/1 -> Product_e2f9b/2
  Constant_x_ddd_31e7b/1 -> Subtract_45c14/1
  Constant_x_l_c31ee/1 -> Subtract_45c14/2
  State_E_fd_SG_D_1_8527f/1 -> Subtract_e067d/1
  Divide_07a74/1 -> Add_9784c/1
  Subtract_e7df9/1 -> Divide_07a74/2
  State_psi_fd_SG_D_1_f98c2/1 -> Product_fd30e/1
  Constant_x_ddd_bc97c/1 -> Divide_e8213/2
  Subtract_45c14/1 -> Product_fd30e/2
  Constant_x_dd_19ab2/1 -> Subtract_2f275/1
  Constant_x_dd_29d28/1 -> Subtract_2df05/1
  State_psi_fd_SG_D_1_d4fb7/1 -> Subtract_e067d/2
  Constant_x_l_dd136/1 -> Subtract_2f275/2
  Product_fd30e/1 -> Divide_b99b5/1
  Constant_-1_f01dd/1 -> Product_e4a4c/1
  Subtract_2f275/1 -> Divide_b99b5/2
  Constant_x_dd_de6c1/1 -> Subtract_2df4e/1
  Add_9784c/1 -> Subtract_e5505/1
  Constant_x_l_79a36/1 -> Subtract_2df05/2
  Divide_b99b5/1 -> Subtract_e5505/2
  Divide_af00d/1 -> Subtract_77a7f/1
  Constant_-1_fa63a/1 -> Product_a6a8b/1
  State_psi_1d_SG_D_1_118f1/1 -> Product_a6a8b/2
  Constant_x_dd_b3c45/1 -> Subtract_d7563/1
  Subtract_35719/1 -> Product_e4a4c/2
  Constant_x_ddd_25389/1 -> Subtract_d7563/2
  Product_a6a8b/1 -> Product_b9875/1
  Constant_2.0_7f266/1 -> Power_57dc6/2
  Product_b9875/1 -> Divide_ce485/1
  Subtract_77a7f/1 -> Product_970ff/2
  Subtract_d7563/1 -> Product_b9875/2
  State_psi_d_SG_D_1_32ce4/1 -> Add_a8ad5/2
  Constant_x_dd_21f9f/1 -> Subtract_d6bf8/1
  Constant_x_l_5df97/1 -> Subtract_d6bf8/2
  Constant_x_dd_f60e6/1 -> Subtract_35719/1
  Divide_e8213/1 -> Subtract_dd92d/2
  Constant_x_ddd_9301e/1 -> Subtract_5bb7f/1
  Constant_x_ddd_08776/1 -> Subtract_35719/2
  Constant_x_l_44d17/1 -> Subtract_5bb7f/2
  Subtract_5bb7f/1 -> Product_ba8f5/2
  State_psi_1d_SG_D_1_7112e/1 -> Subtract_71eff/1
  Product_ba8f5/1 -> Divide_ace08/1
  State_psi_fd_SG_D_1_4440b/1 -> Subtract_71eff/2
  State_psi_fd_SG_D_1_13afa/1 -> Product_ba8f5/1
  Product_b92e4/1 -> Divide_e8213/1
  Divide_ce485/1 -> Add_a8ad5/1
  Subtract_d6bf8/1 -> Divide_ce485/2
  Constant_x_dd_6e386/1 -> Subtract_41cca/1
  Constant_x_l_3f897/1 -> Subtract_41cca/2
  Divide_ace08/1 -> Subtract_baf42/2
  Subtract_71eff/1 -> Subtract_dd92d/1
  Subtract_41cca/1 -> Divide_ace08/2
  Subtract_dd92d/1 -> Product_945d8/2
  Product_e4a4c/1 -> Product_945d8/1
  Subtract_2df05/1 -> Power_57dc6/1
  Add_a8ad5/1 -> Subtract_baf42/1
  Product_945d8/1 -> Divide_af00d/1
  Power_57dc6/1 -> Divide_af00d/2
  Subtract_baf42/1 -> Divide_37f84/1
  Constant_x_ddd_56167/1 -> Divide_37f84/2
  Constant_x_d_c4b24/1 -> Subtract_4c26f/1
  Constant_x_dd_a57e0/1 -> Subtract_4c26f/2
  Divide_37f84/1 -> Subtract_77a7f/2
  Subtract_4c26f/1 -> Product_970ff/1
  Subtract_e067d/1 -> Subtract_04b7e/1
  Product_970ff/1 -> Subtract_04b7e/2
  Subtract_04b7e/1 -> Divide_c873c/1
  Constant_T_dd_aa86a/1 -> Divide_c873c/2
  Divide_c873c/1 -> Blockout_d_psi_fd_SG_D_1_186e8/1

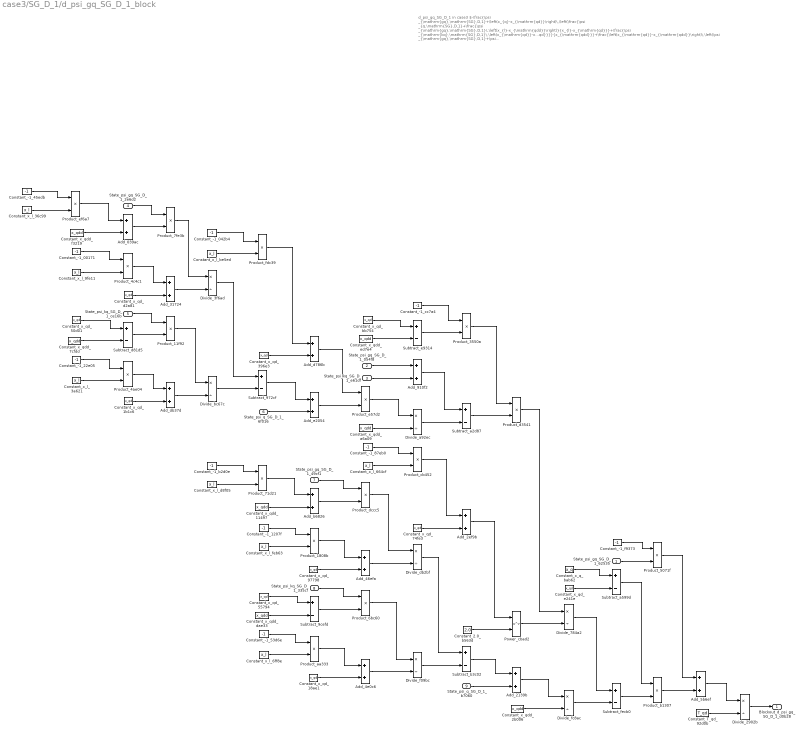
== system case3/SG_D_1/d_psi_gq_SG_D_1_block ==
  note: d_psi_gq_SG_D_1 in case3
      | $-\frac{\psi _{\mathrm{gq},\mathrm{SG},D,1}+\left(x_{q}-x_{\mathrm{qd}}\right)\,\left(\frac{\psi _{q,\mathrm{SG},D,1}+\frac{\psi _{\mathrm{gq},\mathrm{SG},D,1}\,\left(x_{l}-x_{\mathrm{qdd}}\right)}{x_{l}-x_{\mathrm{qd}}}+\frac{\psi _{\mathrm{kq},\mathrm{SG},D,1}\,\left(x_{\mathrm{qd}}-x_{\mathrm{qdd}}\right)}{x_{l}-x_{\mathrm{qd}}}}{x_{\mathrm{qdd}}}+\frac{\left(x_{\mathrm{qd}}-x_{\mathrm{qdd}}\right)\,\left(\psi _{\mathrm{gq},\mathrm{SG},D,1}+\psi _{\mathrm{kq},\mathrm{SG},D,1}+\frac{\left(x_{l}-x_{\mathrm{qd}}\right)\,\left(\psi _{q,\mathrm{SG},D,1}+\frac{\psi _{\mathrm{gq},\mathrm{SG},D,1}\,\left(x_{l}-x_{\mathrm{qdd}}\right)}{x_{l}-x_{\mathrm{qd}}}+\frac{\psi _{\mathrm{kq},\mathrm{SG},D,1}\,\left(x_{\mathrm{qd}}-x_{\mathrm{qdd}}\right)}{x_{l}-x_{\mathrm{qd}}}\right)}{x_{\mathrm{qdd}}}\right)}{{\left(x_{l}-x_{\mathrm{qd}}\right)}^2}\right)}{T_{\mathrm{qd}}}$
      | Automatically generated on 2025-10-31 18:58:59 .
  State_psi_gq_SG_D_1_62535 : Inport
  State_psi_gq_SG_D_1_054f8 : Inport  Port=2
  State_psi_kq_SG_D_1_e61df : Inport  Port=3
  State_psi_gq_SG_D_1_2e6d2 : Inport  Port=4
  State_psi_kq_SG_D_1_ce16b : Inport  Port=5
  State_psi_q_SG_D_1_6f016 : Inport  Port=6
  State_psi_gq_SG_D_1_49cf1 : Inport  Port=7
  State_psi_kq_SG_D_1_335cf : Inport  Port=8
  State_psi_q_SG_D_1_b7060 : Inport  Port=9
  Add_039ac : Sum
  Add_2139b : Sum
  Add_2ef9b : Sum
  Add_31724 : Sum
  Add_46efa : Sum
  Add_4e0c6 : Sum
  Add_5b6ef : Sum
  Add_910f2 : Sum
  Add_b6826 : Sum
  Add_d786b : Sum
  Add_db37d : Sum
  Add_e2054 : Sum
  Constant_-1_00171 : Constant  Value=-1
  Constant_-1_042b4 : Constant  Value=-1
  Constant_-1_1207f : Constant  Value=-1
  Constant_-1_22e05 : Constant  Value=-1
  Constant_-1_45edb : Constant  Value=-1
  Constant_-1_53d6e : Constant  Value=-1
  Constant_-1_87eb0 : Constant  Value=-1
  Constant_-1_b2d0e : Constant  Value=-1
  Constant_-1_cc7a4 : Constant  Value=-1
  Constant_-1_f9373 : Constant  Value=-1
  Constant_2.0_b563d : Constant  Value=2.0
  Constant_T_qd_92d0b : Constant  Value=T_qd
  Constant_x_l_36c99 : Constant  Value=x_l
  Constant_x_l_3a621 : Constant  Value=x_l
  Constant_x_l_664cf : Constant  Value=x_l
  Constant_x_l_6ff8e : Constant  Value=x_l
  Constant_x_l_9fe11 : Constant  Value=x_l
  Constant_x_l_be5ed : Constant  Value=x_l
  Constant_x_l_d8f05 : Constant  Value=x_l
  Constant_x_l_feb63 : Constant  Value=x_l
  Constant_x_q_bab62 : Constant  Value=x_q
  Constant_x_qd_18ae1 : Constant  Value=x_qd
  Constant_x_qd_1b1c6 : Constant  Value=x_qd
  Constant_x_qd_396e3 : Constant  Value=x_qd
  Constant_x_qd_50d01 : Constant  Value=x_qd
  Constant_x_qd_55794 : Constant  Value=x_qd
  Constant_x_qd_74fe3 : Constant  Value=x_qd
  Constant_x_qd_97798 : Constant  Value=x_qd
  Constant_x_qd_bb754 : Constant  Value=x_qd
  Constant_x_qd_d2a81 : Constant  Value=x_qd
  Constant_x_qd_e241e : Constant  Value=x_qd
  Constant_x_qdd_11497 : Constant  Value=x_qdd
  Constant_x_qdd_2b006 : Constant  Value=x_qdd
  Constant_x_qdd_7cfdd : Constant  Value=x_qdd
  Constant_x_qdd_a6a09 : Constant  Value=x_qdd
  Constant_x_qdd_dae33 : Constant  Value=x_qdd
  Constant_x_qdd_ed7e4 : Constant  Value=x_qdd
  Constant_x_qdd_f3219 : Constant  Value=x_qdd
  Divide_2902b : Product  Inputs=*/
  Divide_3f6ad : Product  Inputs=*/
  Divide_784a2 : Product  Inputs=*/
  Divide_a92ec : Product  Inputs=*/
  Divide_bc67c : Product  Inputs=*/
  Divide_db2bf : Product  Inputs=*/
  Divide_f09bc : Product  Inputs=*/
  Divide_fc8ac : Product  Inputs=*/
  Power_cbad2 : Math  Operator=pow
  Product_11f92 : Product
  Product_1808b : Product
  Product_3550a : Product
  Product_4ae04 : Product
  Product_4c4c1 : Product
  Product_5071f : Product
  Product_6bc60 : Product
  Product_71d21 : Product
  Product_7fe3b : Product
  Product_aa333 : Product
  Product_b1307 : Product
  Product_cb452 : Product
  Product_d3541 : Product
  Product_dccc5 : Product
  Product_e57d2 : Product
  Product_ef6a7 : Product
  Product_fdc39 : Product
  Subtract_972cf : Sum  Inputs=+-
  Subtract_9cefd : Sum  Inputs=+-
  Subtract_a2d87 : Sum  Inputs=+-
  Subtract_a599d : Sum  Inputs=+-
  Subtract_b3c02 : Sum  Inputs=+-
  Subtract_d81d5 : Sum  Inputs=+-
  Subtract_e9314 : Sum  Inputs=+-
  Subtract_fecb0 : Sum  Inputs=+-
  Blockout_d_psi_gq_SG_D_1_d0b28 : Outport
  wires:
  State_psi_gq_SG_D_1_2e6d2/1 -> Product_7fe3b/1
  Constant_-1_00171/1 -> Product_4c4c1/1
  Divide_3f6ad/1 -> Subtract_972cf/1
  Add_31724/1 -> Divide_3f6ad/2
  Product_ef6a7/1 -> Add_039ac/1
  Constant_x_qd_396e3/1 -> Add_d786b/2
  Constant_-1_45edb/1 -> Product_ef6a7/1
  Constant_x_qdd_f3219/1 -> Add_039ac/2
  Constant_x_l_9fe11/1 -> Product_4c4c1/2
  Constant_x_l_36c99/1 -> Product_ef6a7/2
  Constant_-1_22e05/1 -> Product_4ae04/1
  Constant_x_qd_50d01/1 -> Subtract_d81d5/1
  Constant_x_qdd_a6a09/1 -> Divide_a92ec/2
  Constant_x_l_3a621/1 -> Product_4ae04/2
  Constant_x_qdd_7cfdd/1 -> Subtract_d81d5/2
  Subtract_972cf/1 -> Add_e2054/1
  Add_039ac/1 -> Product_7fe3b/2
  Product_7fe3b/1 -> Divide_3f6ad/1
  Product_4c4c1/1 -> Add_31724/1
  Constant_x_qd_d2a81/1 -> Add_31724/2
  State_psi_kq_SG_D_1_ce16b/1 -> Product_11f92/1
  Product_4ae04/1 -> Add_db37d/1
  Subtract_d81d5/1 -> Product_11f92/2
  Constant_x_qd_1b1c6/1 -> Add_db37d/2
  Product_11f92/1 -> Divide_bc67c/1
  Add_db37d/1 -> Divide_bc67c/2
  Constant_-1_cc7a4/1 -> Product_3550a/1
  Constant_-1_042b4/1 -> Product_fdc39/1
  Add_46efa/1 -> Divide_db2bf/2
  Product_aa333/1 -> Add_4e0c6/1
  Subtract_9cefd/1 -> Product_6bc60/2
  Constant_x_l_be5ed/1 -> Product_fdc39/2
  Divide_bc67c/1 -> Subtract_972cf/2
  Subtract_a599d/1 -> Product_b1307/1
  Constant_-1_87eb0/1 -> Product_cb452/1
  Constant_-1_b2d0e/1 -> Product_71d21/1
  Constant_x_l_664cf/1 -> Product_cb452/2
  Constant_x_l_d8f05/1 -> Product_71d21/2
  Constant_x_qd_97798/1 -> Add_46efa/2
  Product_fdc39/1 -> Add_d786b/1
  State_psi_q_SG_D_1_6f016/1 -> Add_e2054/2
  Product_71d21/1 -> Add_b6826/1
  Constant_x_qdd_11497/1 -> Add_b6826/2
  Constant_-1_1207f/1 -> Product_1808b/1
  Constant_x_qd_18ae1/1 -> Add_4e0c6/2
  Add_d786b/1 -> Product_e57d2/1
  Constant_x_l_feb63/1 -> Product_1808b/2
  Constant_-1_53d6e/1 -> Product_aa333/1
  Constant_x_qd_55794/1 -> Subtract_9cefd/1
  Product_e57d2/1 -> Divide_a92ec/1
  Constant_x_l_6ff8e/1 -> Product_aa333/2
  Divide_784a2/1 -> Subtract_fecb0/1
  Constant_x_qdd_dae33/1 -> Subtract_9cefd/2
  Add_e2054/1 -> Product_e57d2/2
  State_psi_gq_SG_D_1_49cf1/1 -> Product_dccc5/1
  Add_b6826/1 -> Product_dccc5/2
  Product_1808b/1 -> Add_46efa/1
  State_psi_kq_SG_D_1_335cf/1 -> Product_6bc60/1
  Add_4e0c6/1 -> Divide_f09bc/2
  State_psi_gq_SG_D_1_054f8/1 -> Add_910f2/1
  Constant_x_qd_bb754/1 -> Subtract_e9314/1
  Constant_x_qdd_ed7e4/1 -> Subtract_e9314/2
  Product_6bc60/1 -> Divide_f09bc/1
  State_psi_kq_SG_D_1_e61df/1 -> Add_910f2/2
  Product_dccc5/1 -> Divide_db2bf/1
  Subtract_e9314/1 -> Product_3550a/2
  Add_910f2/1 -> Subtract_a2d87/1
  Divide_a92ec/1 -> Subtract_a2d87/2
  Product_cb452/1 -> Add_2ef9b/1
  Constant_x_qd_74fe3/1 -> Add_2ef9b/2
  Divide_db2bf/1 -> Subtract_b3c02/1
  Divide_f09bc/1 -> Subtract_b3c02/2
  Product_3550a/1 -> Product_d3541/1
  Subtract_a2d87/1 -> Product_d3541/2
  Add_2ef9b/1 -> Power_cbad2/1
  Constant_2.0_b563d/1 -> Power_cbad2/2
  Subtract_b3c02/1 -> Add_2139b/1
  State_psi_q_SG_D_1_b7060/1 -> Add_2139b/2
  Product_d3541/1 -> Divide_784a2/1
  Power_cbad2/1 -> Divide_784a2/2
  Add_2139b/1 -> Divide_fc8ac/1
  Constant_x_qdd_2b006/1 -> Divide_fc8ac/2
  Constant_x_q_bab62/1 -> Subtract_a599d/1
  Constant_x_qd_e241e/1 -> Subtract_a599d/2
  Divide_fc8ac/1 -> Subtract_fecb0/2
  Constant_-1_f9373/1 -> Product_5071f/1
  State_psi_gq_SG_D_1_62535/1 -> Product_5071f/2
  Subtract_fecb0/1 -> Product_b1307/2
  Product_5071f/1 -> Add_5b6ef/1
  Product_b1307/1 -> Add_5b6ef/2
  Add_5b6ef/1 -> Divide_2902b/1
  Constant_T_qd_92d0b/1 -> Divide_2902b/2
  Divide_2902b/1 -> Blockout_d_psi_gq_SG_D_1_d0b28/1
